simulink model "TestAssignmentImplementingUnitTime"  (R2017b)
settings: Solver=VariableStepAuto  StartTime=0.0  StopTime=100  FixedStep=1  MaxStep=1  RelTol=1e-3
undefined symbols (not defined in the file): ok
settings Model: Creator=georgimarkov  LastModifiedBy=georgimarkov

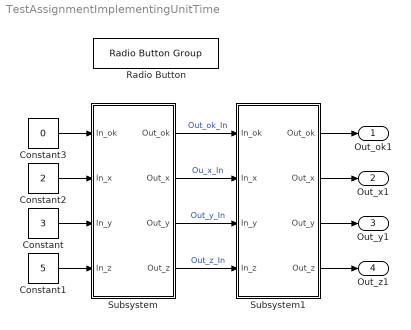
== system TestAssignmentImplementingUnitTime ==
  Constant : Constant  Value=3
  Constant1 : Constant  Value=5
  Constant2 : Constant  Value=2
  Constant3 : Constant  Value=0
  Radio Button : RadioButtonGroup  WebBlockId=85  ModelName=TestAssignmentImplementingUnitTime  LabelPosition=Top  ShowInitialText=on  SelectedLabel=-ok  ButtonGroupName=Group
      settings: Values={{'-ok', 'ok'}, [0 1]}
  Subsystem : Subsystem
  Subsystem1 : Subsystem
  Out_ok1 : Outport
  Out_x1 : Outport  Port=2
  Out_y1 : Outport  Port=3
  Out_z1 : Outport  Port=4
  wires:
  Constant3/1 -> Subsystem/1(In_ok)
  Constant2/1 -> Subsystem/2(In_x)
  Constant/1 -> Subsystem/3(In_y)
  Constant1/1 -> Subsystem/4(In_z)
  Subsystem/2(Out_x) -> Subsystem1/2(In_x)  "Ou_x_In"
  Subsystem1/4(Out_z) -> Out_z1/1
  Subsystem1/1(Out_ok) -> Out_ok1/1
  Subsystem1/2(Out_x) -> Out_x1/1
  Subsystem/3(Out_y) -> Subsystem1/3(In_y)  "Out_y_In"
  Subsystem/4(Out_z) -> Subsystem1/4(In_z)  "Out_z_In"
  Subsystem/1(Out_ok) -> Subsystem1/1(In_ok)  "Out_ok_In"
  Subsystem1/3(Out_y) -> Out_y1/1

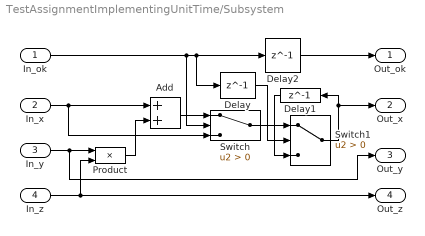
== system TestAssignmentImplementingUnitTime/Subsystem ==
  In_ok : Inport
  In_x : Inport  Port=2
  In_y : Inport  Port=3
  In_z : Inport  Port=4
  Add : Sum
  Delay : Delay  DelayLength=1  InitialCondition=0
  Delay1 : Delay  DelayLength=1  InitialCondition=0
  Delay2 : Delay  DelayLength=1  InitialCondition=0
  Product : Product
  Switch : Switch  Criteria=u2 > Threshold
  Switch1 : Switch  Criteria=u2 > Threshold
  Out_ok : Outport
  Out_x : Outport  Port=2
  Out_y : Outport  Port=3
  Out_z : Outport  Port=4
  wires:
  In_y/1 -> Out_y/1, Product/1
  Delay1/1 -> Switch1/1
  Switch1/1 -> Out_x/1, Delay1/1
  In_x/1 -> Switch/3, Add/1
  In_z/1 -> Out_z/1, Product/2
  Switch/1 -> Switch1/3
  Delay/1 -> Switch1/2
  In_ok/1 -> Delay2/1, Delay/1, Switch/2
  Product/1 -> Add/2
  Add/1 -> Switch/1
  Delay2/1 -> Out_ok/1

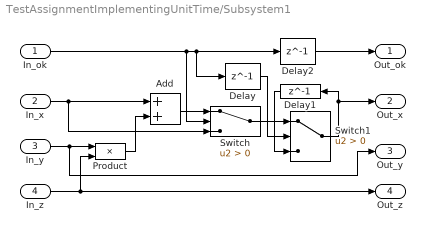
== system TestAssignmentImplementingUnitTime/Subsystem1 ==
  In_ok : Inport
  In_x : Inport  Port=2
  In_y : Inport  Port=3
  In_z : Inport  Port=4
  Add : Sum
  Delay : Delay  DelayLength=1  InitialCondition=0
  Delay1 : Delay  DelayLength=1  InitialCondition=0
  Delay2 : Delay  DelayLength=1  InitialCondition=0
  Product : Product
  Switch : Switch  Criteria=u2 > Threshold
  Switch1 : Switch  Criteria=u2 > Threshold
  Out_ok : Outport
  Out_x : Outport  Port=2
  Out_y : Outport  Port=3
  Out_z : Outport  Port=4
  wires:
  In_y/1 -> Out_y/1, Product/1
  Delay1/1 -> Switch1/1
  Switch1/1 -> Out_x/1, Delay1/1
  In_x/1 -> Switch/3, Add/1
  In_z/1 -> Out_z/1, Product/2
  Switch/1 -> Switch1/3
  Delay/1 -> Switch1/2
  In_ok/1 -> Delay2/1, Delay/1, Switch/2
  Product/1 -> Add/2
  Add/1 -> Switch/1
  Delay2/1 -> Out_ok/1
